simulink model "symulacja_zapisplik"  (R2017b)
settings: Solver=VariableStepAuto  StartTime=0.0  StopTime=10.0  RelTol=1e-3
values from neighbouring files (symbols this model uses):
  FV = 1    [projekt2.m]
  K = 1.4    [projekt2.m]
  T1 = 1/14    (= 0.0714285714286)    [projekt2.m]
  T2 = 100    [projekt2.m]
  T3 = 10    [projekt2.m]
  T4 = 1    [projekt2.m]
settings Model: Creator=Alicja  LastModifiedBy=Alicja

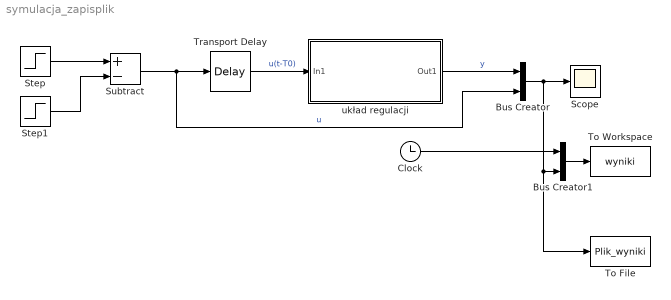
== system symulacja_zapisplik ==
  Bus Creator : BusCreator  Inputs=2
  Bus Creator1 : BusCreator  Inputs=2
  Clock : Clock
  Scope : Scope
  Step : Step  Time=10  SampleTime=0
  Step1 : Step  Time=11  After=FV  SampleTime=0
  Subtract : Sum  Inputs=+-
  To File : ToFile  Filename=Plik_wyniki  MatrixName=sim_wyniki
  To Workspace : ToWorkspace  VariableName=wyniki  SampleTime=-1
  Transport Delay : TransportDelay  DelayTime=20
  układ regulacji : Subsystem
  wires:
  Bus Creator/1 -> Bus Creator1/2, To File/1, Scope/1
  Transport Delay/1 -> układ regulacji/1(In1)  "u(t-T0)"
  układ regulacji/1(Out1) -> Bus Creator/1  "y"
  Subtract/1 -> Transport Delay/1, Bus Creator/2  "u"
  Step/1 -> Subtract/1
  Step1/1 -> Subtract/2
  Bus Creator1/1 -> To Workspace/1
  Clock/1 -> Bus Creator1/1

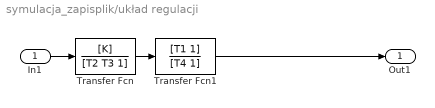
== system symulacja_zapisplik/układ regulacji ==
  In1 : Inport
  Transfer Fcn : TransferFcn  Numerator=[K]  Denominator=[T2 T3 1]
  Transfer Fcn1 : TransferFcn  Numerator=[T1 1]  Denominator=[T4 1]
  Out1 : Outport
  wires:
  Transfer Fcn/1 -> Transfer Fcn1/1
  In1/1 -> Transfer Fcn/1
  Transfer Fcn1/1 -> Out1/1
